simulink model "M10B39_es_V3"  (R2025a)
settings: Solver=ode23tb  StartTime=0.0  StopTime=100  FixedStep=0.001  MaxStep=0.01  RelTol=1e-3  EnableMultiTasking=on
InitFcn:
  | initAll_V3
values from neighbouring files (symbols this model uses):
  acom = 100    [initAll_V1.m]    (also in initAll_V2.m; initAll_V3.m; parameterinit.mat)
  AVm0 = [4.26082678503 4.656135219]    [parameterinit.mat]
  bcom = 50    [initAll_V1.m]    (also in initAll_V2.m; initAll_V3.m; parameterinit.mat)
  commun = 0*commun    [initAll_V1.m]    (also in initAll_V2.m; initAll_V3.m; parameterinit.mat = [0  0  0; 0  0  0; 0  0  0; 0  0  0])
  DataDelay = 0.0*DataDelay    [initAll_V1.m]    (also in initAll_V2.m; initAll_V3.m; parameterinit.mat = [0  0  0; 0  0  0; 0  0  0; 0  0  0])
  ESinit =     [parameterinit.mat]
  fB = 50    [initAll.m]    (also in initAll_V1.m; initAll_V2.m; initAll_V3.m; parameterinit.mat)
  Geninit = Generator_init(opdata,SynMach_in_gidx)    [initAll.m]    (also in initAll_V1.m; initAll_V2.m; initAll_V3.m = Generator_init(opdata_all,SynMach_in_gidx1); parameterinit.mat = )
  lam = 100    [initAll_V1.m]    (also in initAll_V2.m; initAll_V3.m; parameterinit.mat)
  SgridB = 100    [initAll.m]    (also in initAll_V1.m; initAll_V2.m; initAll_V3.m; parameterinit.mat)
  wB = 2*pi*fB    (= 314.159265359)    [initAll.m]    (also in initAll_V1.m; initAll_V2.m; initAll_V3.m; parameterinit.mat)
  Windinit =     [parameterinit.mat]
  YY_load = [3.65450097002 -2.05705688056 0 0 0 0 0 0 0 0 0 0 ... (1521 elements, 39x39)]    [parameterinit.mat]    (also in powerflowcaculate.m = full(YY))
undefined symbols (not defined in the file or in its folder): c1, c2, c3, c4, c5, c6, cp_nom, lambda_nom, P_wind_base, Pelec_base, Pnom
libraries: spsBistableLib x12, simulink_extras x3, slpidlib x2, simulink x1
(part 5 of 7)

== system M10B39_es_V3/Genrators/Wind Generator - DFIG1/Asynchronous Machine Equations  ==
  note: Vsdq
  s / ω_B : Inport
  Vgxy : Inport  Port=2
  Vrxy : Inport  Port=3
  "Trip " : Inport  Port=4
  3th order Transient Equations : Subsystem
  Add : Sum  Inputs=+-
  Constant : Constant  Value=Za
  Constant1 : Constant  Value=0
  Fcn6 : Fcn  Expr=sqrt(u(1)^2+u(2)^2)
  Gain2 : Gain  Gain=NPf
  Interface : Subsystem
  Multiply : Product  Multiplication=Matrix(*)
  Mux2 : Mux  Inputs=2
  Mux4 : Mux  Inputs=2
  Ps_ : Fcn  Expr=u(1)*u(3)+u(2)*u(4)
  Qs_ : Fcn  Expr=u(2)*u(3)-u(1)*u(4)
  Scope : Scope
      settings: ActiveDisplayYMinimum=-0.69793  ActiveDisplayYMaximum=9.95802
  Scope1 : Scope
      settings: ActiveDisplayYMinimum=0.89985  ActiveDisplayYMaximum=1.09985
  Selector : Selector  InputPortWidth=2  IndexOptions=Index vector (dialog)  Indices=[2 1]  OutputSizes=1
  Te_ : Fcn  Expr=u(2)*u(3)+u(1)*u(4)
  Te : Outport
  Ps : Outport  Port=2
  Qs : Outport  Port=3
  Irxy : Outport  Port=4
  Exy : Outport  Port=5
  Isxy1 : Outport  Port=6
  GBxy : Outport  Port=7
  wires:
  "Trip "/1 -> 3th order Transient Equations/4(Trip)
  3th order Transient Equations/1(Irxy) -> Irxy/1
  Qs_/1 -> Qs/1, Scope/1
  Constant1/1 -> Interface/1(delta)
  Gain2/1 -> Te/1
  Vgxy/1 -> Add/1, Fcn6/1, Mux2/1
  Add/1 -> Multiply/2
  Constant/1 -> Multiply/1
  Selector/1 -> Exy/1, Add/2
  Te_/1 -> Gain2/1
  Mux4/1 -> Te_/1
  s / ω_B/1 -> 3th order Transient Equations/3(s / ω_B)
  Ps_/1 -> Ps/1
  Interface/1(Igxy1) -> Isxy1/1
  Interface/2(GBxy) -> GBxy/1
  Mux2/1 -> Qs_/1, Ps_/1
  Vrxy/1 -> 3th order Transient Equations/2(Vrxy)
  Multiply/1 -> 3th order Transient Equations/1(Isxy), Mux4/1, Mux2/2
  Fcn6/1 -> Scope1/1
  3th order Transient Equations/2(Eyx) -> Mux4/2, Selector/1, Interface/2(Eqd)

== system M10B39_es_V3/Genrators/Wind Generator - DFIG1/Converter function ==
  Vsxy : Inport
  Vcxy : Inport  Port=2
  Trip : Inport  Port=3
  Change_choke : Gain  Gain=[1 -1]  SaturateOnIntegerOverflow=on  OutDataTypeStr=Inherit: Same as input  ParamDataTypeStr=Inherit: Same as input
  Constant2 : Constant  Value=0
  GSC_Idq : Integrator  InitialCondition=[Icx0 Icy0]
  L_choke : Gain  Gain=Lg  SaturateOnIntegerOverflow=on  OutDataTypeStr=Inherit: Same as input  ParamDataTypeStr=Inherit: Same as input
  R_choke : Gain  Gain=Rg  SaturateOnIntegerOverflow=on  OutDataTypeStr=Inherit: Same as input  ParamDataTypeStr=Inherit: Same as input
  Selector : Selector  InputPortWidth=2  IndexOptions=Index vector (dialog)  Indices=[2 1]  OutputSizes=1
  Sum : Sum  Inputs=+--+  SaturateOnIntegerOverflow=on
  Switch1 : Switch  Criteria=u2 ~= 0  Threshold=0.5  InputSameDT=off
  Switch4 : Switch  Criteria=u2 ~= 0  Threshold=0.5  InputSameDT=off
  W/L : Gain  Gain=wB / Lg  SaturateOnIntegerOverflow=on  OutDataTypeStr=Inherit: Same as input  ParamDataTypeStr=Inherit: Same as input
  Ixy_gsc : Outport
  wires:
  Switch4/1 -> Ixy_gsc/1, R_choke/1, Selector/1
  GSC_Idq/1 -> Switch4/3
  Switch1/1 -> GSC_Idq/1
  W/L/1 -> Switch1/3
  Constant2/1 -> Switch4/1, Switch1/1
  Trip/1 -> Switch1/2, Switch4/2
  Vcxy/1 -> Sum/2
  Change_choke/1 -> Sum/4
  Sum/1 -> W/L/1
  R_choke/1 -> Sum/3
  Vsxy/1 -> Sum/1
  Selector/1 -> L_choke/1
  L_choke/1 -> Change_choke/1

== system M10B39_es_V3/Genrators/Wind Generator - DFIG1/DC Bus model ==
  note: Pdc = Pr_gsc - Pr_rsc
  Pr_gsc : Inport
  Pr_rsc : Inport  Port=2
  Product2 : Product  Inputs=*/  InputSameDT=on  SaturateOnIntegerOverflow=on  OutDataTypeStr=Inherit: Same as first input
  Sum2 : Sum  Inputs=+-  InputSameDT=on  SaturateOnIntegerOverflow=on  OutDataTypeStr=Inherit: Same as first input
  Udc : Integrator  InitialCondition=Vdc0  LowerSaturationLimit=1e-6  ZeroCross=off
  deg->rad1 : Gain  Gain=1/C_w  SaturateOnIntegerOverflow=on  OutDataTypeStr=Inherit: Same as input  ParamDataTypeStr=Inherit: Same as input
  deg->rad2 : Gain  Gain=wB  SaturateOnIntegerOverflow=on  OutDataTypeStr=Inherit: Same as input  ParamDataTypeStr=Inherit: Same as input
  Vdc : Outport
  wires:
  deg->rad2/1 -> deg->rad1/1
  Sum2/1 -> Product2/1
  deg->rad1/1 -> Udc/1
  Pr_gsc/1 -> Sum2/1
  Product2/1 -> deg->rad2/1  "Idc"
  Udc/1 -> Product2/2, Vdc/1  "Vdc"
  Pr_rsc/1 -> Sum2/2

== system M10B39_es_V3/Genrators/Wind Generator - DFIG1/Grid Side Converter and control ==
  note: K为系数，p/i为系数的名字，DC/Id/Iq为控制的量，g为GSC，w为wind，与直流电网的VSC参数区分开来
  Vdc : Inport
  Vsdq : Inport  Port=2
  Icdq : Inport  Port=3
  Enable : EnablePort
  Add : Sum  Inputs=|+-
  Add{1,3,5,7,11} (5 alike) : Sum
  Add10 : Sum  Commented=on
  Add2 : Sum  Inputs=|+-
  Add4 : Sum  Inputs=|-+
  Add6 : Sum  Inputs=|+-
  Add8 : Sum  Inputs=|-+
  Add9 : Sum  Inputs=-+
  Constant : Constant  Value=Vdc_w
  Constant1 : Constant  Value=Icq_ref
  Constant2 : Constant
  Demux : Demux  Outputs=2
  Demux1 : Demux  Outputs=2
  From12 : From  Commented=on  GotoTag=Icd
  From13 : From  Commented=on  GotoTag=Icq
  From14 : From  Commented=on  GotoTag=Ucd
  From15 : From  Commented=on  GotoTag=Ucq
  Gain : Gain  Gain=KpDC_gw
  Gain1 : Gain  Gain=KiDC_gw
  Gain2 : Gain  Gain=KpId_gw
  Gain3 : Gain  Gain=KiId_gw
  Gain4 : Gain  Gain=Lg
  Gain5 : Gain  Gain=KpIq_gw
  Gain6 : Gain  Gain=KiIq_gw
  Gain7 : Gain  Gain=Lg
  KiDC_gw : Integrator  InitialCondition=Icd_ref
  KiId_gw : Integrator
  KiIq_gw : Integrator
  Multiply{,1,4..5} (4 alike) : Product
  Multiply2 : Product  Commented=on
  Multiply3 : Product  Commented=on
  Mux : Mux  Inputs=2
  Scope1 : Scope
      settings: ActiveDisplayYMinimum=0.114016671  ActiveDisplayYMaximum=0.114016689  DataLoggingVariableName=ScopeData4
  Scope3 : Scope
      settings: ActiveDisplayYMinimum=-1.4E-17  ActiveDisplayYMaximum=9E-18  DataLoggingVariableName=ScopeData11
  Scope4 : Scope
      settings: ActiveDisplayYMinimum=-0.04026  ActiveDisplayYMaximum=0.20394  DataLoggingVariableName=ScopeData12
  Pr_gsc : Outport
  ucdq : Outport  Port=2
  wires:
  Demux1/2 -> [Icq]
  Icdq/1 -> Demux1/1
  Demux1/1 -> [Icd]
  Mux/1 -> ucdq/1
  Add8/1 -> Mux/2
  Add4/1 -> Mux/1
  Add6/1 -> Gain5/1, Gain6/1, Scope3/1
  Add11/1 -> Pr_gsc/1
  Multiply5/1 -> Add11/2
  Multiply4/1 -> Add11/1
  [Vsd] -> Multiply4/1
  [Vsq] -> Multiply5/1
  [Icd] -> Multiply4/2
  [Icq] -> Multiply5/2
  From14/1 -> Multiply2/1
  From12/1 -> Multiply2/2
  Multiply2/1 -> Add10/1
  From15/1 -> Multiply3/1
  From13/1 -> Multiply3/2
  Multiply3/1 -> Add10/2
  Add9/1 -> Add8/2
  Multiply1/1 -> Gain7/1
  [Icd] -> Multiply1/2
  Gain7/1 -> Add9/1
  [Vsq] -> Add9/2
  [We] -> Multiply1/1
  Gain6/1 -> KiIq_gw/1
  Gain5/1 -> Add7/1
  KiIq_gw/1 -> Add7/2
  Add7/1 -> Add8/1  "Vgq'"
  Constant1/1 -> Add6/1
  [Icq] -> Add6/2
  [Vsd] -> Add5/2
  Demux/1 -> [Vsd]
  Demux/2 -> [Vsq]
  Vsdq/1 -> Demux/1, [Vsdq]
  Add5/1 -> Add4/2
  Gain4/1 -> Add5/1
  [Icq] -> Multiply/2
  Multiply/1 -> Gain4/1
  [We] -> Multiply/1
  Add3/1 -> Add4/1  "Vgd'"
  Gain3/1 -> KiId_gw/1
  KiId_gw/1 -> Add3/2
  Add2/1 -> Gain2/1, Gain3/1, Scope4/1
  Gain2/1 -> Add3/1
  [Icd] -> Add2/2, Scope1/1
  Add1/1 -> Add2/1  "Iref_cd*"
  KiDC_gw/1 -> Add1/2
  Gain1/1 -> KiDC_gw/1
  Gain/1 -> Add1/1
  Add/1 -> Gain/1, Gain1/1
  [Vdc] -> Add/2
  Constant/1 -> Add/1
  Constant2/1 -> [We]
  Vdc/1 -> [Vdc]

== system M10B39_es_V3/Genrators/Wind Generator - DFIG1/Mechanical DE ==
  note: 这里是电动机惯例，因此发电的时候力矩应该是负的
  note: $\frac{d\omega_r}{dt}=\frac{1}{H}(T_e-T_m)$
      | 电动机惯例
  Te : Inport
  Tm : Inport  Port=2
  AWr : Integrator  InitialCondition=Wr0
  Add : Sum  Inputs=+-
  Constant2 : Constant
  Gain : Gain  Gain=1/H
  Scope : Scope
      settings: ActiveDisplayYMinimum=0.89006  ActiveDisplayYMaximum=0.98946
  Scope2 : Scope
      settings: ActiveDisplayYMinimum=-0.25  ActiveDisplayYMaximum=2.25  DataLoggingVariableName=ScopeData4
  Sum : Sum  Inputs=|-+
  "s " : Outport
  Wr : Outport  Port=2
  wires:
  Sum/1 -> "s "/1
  Tm/1 -> Scope2/1, Add/2
  Add/1 -> Gain/1
  Constant2/1 -> Sum/2
  Gain/1 -> AWr/1
  Te/1 -> Add/1
  AWr/1 -> Sum/1, Wr/1, Scope/1

== system M10B39_es_V3/Genrators/Wind Generator - DFIG1/NoIdealPLL ==
  note: $-V_{x}*sin(\delta_{pcc})+V_{y}*cos(\delta_{pcc})$
  Vsxy : Inport
  Add : Sum
  Add1 : Sum
  Constant : Constant
  Fcn1 : Fcn  Expr=sqrt(u(1)*u(1)+u(2)*u(2))
  Fcn3 : Fcn  Expr=u(1)*cos(u(3))+u(2)*sin(u(3))
  Fcn4 : Fcn  Expr=-u(1)*sin(u(3))+u(2)*cos(u(3))
  Gain : Gain  Gain=Kppll
  Gain1 : Gain  Gain=Kipll
  Integrator : Integrator
  Mux1 : Mux  Inputs=2
  Mux4 : Mux  Inputs=2
  PLL : Integrator  InitialCondition=Atheta
  Scope{,1..3} (4 alike) : Scope
      Scope settings: ActiveDisplayYMinimum=-0.99937  ActiveDisplayYMaximum=8.99437
      Scope1 settings: ActiveDisplayYMinimum=0.98212  ActiveDisplayYMaximum=1.13956
      Scope2 settings: ActiveDisplayYMinimum=0.98677  ActiveDisplayYMaximum=1.11907  DataLoggingVariableName=ScopeData2
      Scope3 settings: ActiveDisplayYMinimum=0.99657  ActiveDisplayYMaximum=1.01572
  low pass filter : simulink_extras/Additional Linear/Transfer Fcn (with initial outputs)  N=[1]  D="[1e-1  1]"  Y0=1  U0=1
  Vsdq : Outport
  Atheta : Outport  Port=2
  fw : Outport  Port=3
  wires:
  Fcn1/1 -> Scope3/1
  Add1/1 -> PLL/1, Add/1
  Fcn4/1 -> Mux1/2, Gain1/1, Gain/1
  Gain1/1 -> Integrator/1
  Integrator/1 -> Add1/2
  Gain/1 -> Add1/1
  low pass filter/1 -> fw/1, Scope2/1
  Add/1 -> low pass filter/1, Scope1/1
  Constant/1 -> Add/2
  Fcn3/1 -> Mux1/1
  Vsxy/1 -> Mux4/1
  Mux1/1 -> Vsdq/1, Fcn1/1
  Mux4/1 -> Fcn4/1, Fcn3/1
  PLL/1 -> Scope/1, Atheta/1, Mux4/2

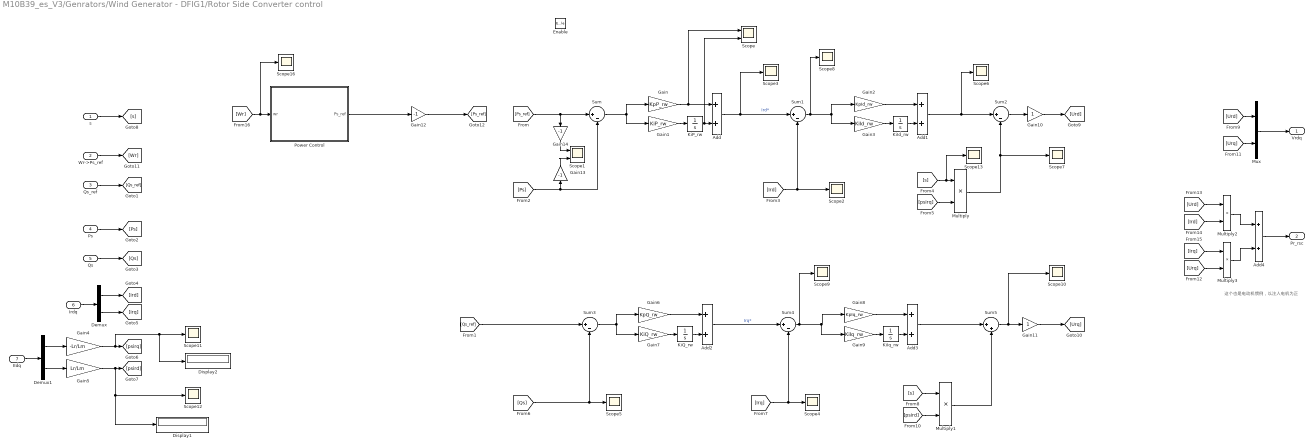
== system M10B39_es_V3/Genrators/Wind Generator - DFIG1/Rotor Side Converter control ==
  note: 这个也是电动机惯例，以注入电机为正
  s : Inport
  Wr->Ps_ref : Inport  Port=2
  Qs_ref : Inport  Port=3
  Ps : Inport  Port=4
  Qs : Inport  Port=5
  Irdq : Inport  Port=6
  Edq : Inport  Port=7
  Enable : EnablePort
  Add{,1..4} (5 alike) : Sum
  Demux : Demux  Outputs=2
  Demux1 : Demux  Outputs=2
  Display1 : Display
  Display2 : Display
  Gain : Gain  Gain=KpP_rw
  Gain1 : Gain  Gain=KiP_rw
  Gain10 : Gain
  Gain11 : Gain
  Gain12 : Gain  Gain=-1
  Gain13 : Gain  Gain=-1
  Gain14 : Gain  Gain=-1
  Gain2 : Gain  Gain=KpId_rw
  Gain3 : Gain  Gain=KiId_rw
  Gain4 : Gain  Gain=-Lr/Lm
  Gain5 : Gain  Gain=Lr/Lm
  Gain6 : Gain  Gain=KpQ_rw
  Gain7 : Gain  Gain=KiQ_rw
  Gain8 : Gain  Gain=KpIq_rw
  Gain9 : Gain  Gain=KiIq_rw
  KiId_rw : Integrator
  KiIq_rw : Integrator
  KiP_rw : Integrator  InitialCondition=Ird_ref
  KiQ_rw : Integrator  InitialCondition=Irq_ref
  Multiply{,1..3} (4 alike) : Product
  Mux : Mux  Inputs=2
  Power Control : Subsystem
  Scope : Scope  NumInputPorts=2
      settings: ActiveDisplayYMinimum=-0.15787  ActiveDisplayYMaximum=1.4048
  Scope1 : Scope  NumInputPorts=2
      settings: ActiveDisplayYMinimum=0.941157  ActiveDisplayYMaximum=0.94124  DataLoggingVariableName=ScopeData2
  Scope{2..13,16} (13 alike) : Scope
      Scope10 settings: ActiveDisplayYMinimum=-0.02713  ActiveDisplayYMaximum=0.00724  DataLoggingVariableName=ScopeData10
      Scope11 settings: DataLoggingVariableName=ScopeData13
      Scope12 settings: DataLoggingVariableName=ScopeData14
      Scope13 settings: ActiveDisplayYMinimum=-0.23407  ActiveDisplayYMaximum=0.19201  DataLoggingVariableName=ScopeData15
      Scope16 settings: ActiveDisplayYMinimum=-1.125  ActiveDisplayYMaximum=0.125  DataLoggingVariableName=ScopeData2
      Scope2 settings: ActiveDisplayYMinimum=0.9164  ActiveDisplayYMaximum=0.98721  DataLoggingVariableName=ScopeData4
      Scope3 settings: ActiveDisplayYMinimum=1.1610912356  ActiveDisplayYMaximum=1.1610912369  DataLoggingVariableName=ScopeData5
      Scope4 settings: ActiveDisplayYMinimum=-0.86275  ActiveDisplayYMaximum=6.60838  DataLoggingVariableName=ScopeData2
      Scope5 settings: ActiveDisplayYMinimum=-8E-13  ActiveDisplayYMaximum=6E-13  DataLoggingVariableName=ScopeData3
      Scope6 settings: ActiveDisplayYMinimum=0.00428  ActiveDisplayYMaximum=0.05974  DataLoggingVariableName=ScopeData2
      Scope7 settings: ActiveDisplayYMinimum=-0.10258  ActiveDisplayYMaximum=-0.10236  DataLoggingVariableName=ScopeData3
      Scope8 settings: ActiveDisplayYMinimum=-0.15319  ActiveDisplayYMaximum=1.32201  DataLoggingVariableName=ScopeData4
      Scope9 settings: ActiveDisplayYMinimum=-0.42548  ActiveDisplayYMaximum=0.04779  DataLoggingVariableName=ScopeData9
  Sum{,1..4} (5 alike) : Sum  Inputs=|+-
  Sum5 : Sum  Inputs=|++
  Vrdq : Outport
  Pr_rsc : Outport  Port=2
  wires:
  Gain12/1 -> [Ps_ref]
  Gain13/1 -> Scope1/2
  Gain14/1 -> Scope1/1
  [Qs_ref] -> Sum3/1
  Power Control/1(Ps_ref) -> Gain12/1
  [Wr] -> Power Control/1(wr), Scope16/1
  [Ird] -> Sum1/2, Scope2/1
  Add4/1 -> Pr_rsc/1
  Multiply3/1 -> Add4/2
  Multiply2/1 -> Add4/1
  [Urq] -> Multiply3/2
  [Irq] -> Multiply3/1
  [Ird] -> Multiply2/2
  [Urd] -> Multiply2/1
  KiP_rw/1 -> Add/2, Scope/2
  Gain/1 -> Add/1, Scope/1
  Gain11/1 -> [Urq]
  Gain10/1 -> [Urd]
  Mux/1 -> Vrdq/1
  [Urq] -> Mux/2
  [Urd] -> Mux/1
  Sum5/1 -> Gain11/1, Scope10/1
  Multiply1/1 -> Sum5/2
  [psird] -> Multiply1/2
  [s] -> Multiply1/1
  Add3/1 -> Sum5/1
  Gain9/1 -> KiIq_rw/1
  Sum4/1 -> Gain8/1, Gain9/1, Scope9/1
  Gain8/1 -> Add3/1
  KiIq_rw/1 -> Add3/2
  [Irq] -> Sum4/2, Scope4/1
  Gain7/1 -> KiQ_rw/1
  KiQ_rw/1 -> Add2/2
  Gain6/1 -> Add2/1
  Sum3/1 -> Gain6/1, Gain7/1
  Add2/1 -> Sum4/1  "Irq*"
  [Qs] -> Sum3/2, Scope5/1
  Sum2/1 -> Gain10/1
  Multiply/1 -> Sum2/2, Scope7/1
  [psirq] -> Multiply/2
  [s] -> Multiply/1, Scope13/1
  Gain5/1 -> [psird], Display1/1, Scope12/1
  Gain4/1 -> [psirq], Scope11/1, Display2/1
  Demux1/1 -> Gain4/1
  s/1 -> [s]
  Edq/1 -> Demux1/1
  Demux1/2 -> Gain5/1
  Gain3/1 -> KiId_rw/1
  KiId_rw/1 -> Add1/2
  Gain2/1 -> Add1/1
  Sum1/1 -> Gain2/1, Gain3/1, Scope8/1
  Add1/1 -> Sum2/1, Scope6/1
  Add/1 -> Scope3/1, Sum1/1  "Ird*"
  Sum/1 -> Gain/1, Gain1/1
  Gain1/1 -> KiP_rw/1
  [Ps] -> Gain13/1, Sum/2
  [Ps_ref] -> Sum/1, Gain14/1
  Demux/2 -> [Irq]
  Demux/1 -> [Ird]
  Irdq/1 -> Demux/1
  Qs/1 -> [Qs]
  Ps/1 -> [Ps]
  Qs_ref/1 -> [Qs_ref]
  Wr->Ps_ref/1 -> [Wr]

== system M10B39_es_V3/Genrators/Wind Generator - DFIG1/Wind Turbine ==
  note: $C_p=0.22* \lbrack 116*(\frac{1}{\lambda+0.008\beta}-\frac{0.0035}{\beta^3+1})-0.48\beta-5 \rbrack * e^{-12.5*(\frac{1}{\lambda+0.08\beta}-\frac{0.035}{\beta^3+1}) }$
  note: $P_m=0.95*\frac{1.2}{(12^3*0.5)}*\lbrack 43.268*(\frac{v_w}{99.4945*\omega_r}-0.035)-1.865 \rbrack * e^{-12.5*(\frac{v_w}{99.4945*\omega_r}-0.035) }*v_w^3$
  note: $C_p= \lbrack 43.268*(\frac{v_w}{99.4945*\omega_r}-0.035)-1.865 \rbrack * e^{-12.5*(\frac{v_w}{99.4945*\omega_r}-0.035) }$
  note: $P_m=0.95*\frac{1.2}{(12^3*0.5)}*\lbrack 43.268*(\frac{1}{99.4945*\frac{\omega_r}{v_w}}-0.035)-1.865 \rbrack * e^{-12.5*(\frac{1}{99.4945*\frac{\omega_r}{v_w}}-0.035) }*v_w^3$
  note: $C_p= \lbrack 43.268*(\frac{1}{99.4945*\frac{\omega_r}{v_w}}-0.035)-1.865 \rbrack * e^{-12.5*(\frac{1}{99.4945*\frac{\omega_r}{v_w}}-0.035) }$
  note: $P_m=0.95*\frac{1.2}{(12^3*0.5)}*C_p*v_w^3$
  note: $C_p= \lbrack 43.268*(\frac{1}{\lambda}-0.035)-1.865 \rbrack * e^{-12.5*(\frac{1}{\lambda}-0.035) }$
  note: $C_p=0.373* \lbrack 116*(\frac{1}{\lambda}-0.035)-5 \rbrack * e^{-12.5*(\frac{1}{\lambda}-0.035) }$
  note: 叶片旋转角速度
  note: 风力机输出
      | 的机械功率
  note: 叶尖速比
  note: 风能利用系数与桨矩角
      | 和叶尖速比之间的关系
  note: 风能利用
      | 系数
  note: 风力机输出
      | 的机械功率
  note: 风速
  note: 叶片旋转速度
  note: 考虑了机械损耗
  note: $\lambda=99.4945*\frac{\omega_r}{v_w}$
  note: $C_p=0.373* \lbrack 116*(\frac{1}{\lambda+0.08\beta}-\frac{0.035}{\beta^3+1})-0.4\beta-5 \rbrack * e^{-12.5*(\frac{1}{\lambda+0.08\beta}-\frac{0.035}{\beta^3+1}) }$
  note: $P_m=\frac{1.2}{(12^3*0.5)}*C_p*v_w^3$
  note: J. Chen and D. Jiang, "Study on modeling and simulation of non-grid-connected wind turbine," 2009 World Non-Grid-Connected Wind Power and Energy Conference , Nanjing, 2009, pp. 1-5. doi: 10.1109/WNWEC.2009.5335791
  W_wt (pu) : Inport
  Pitch angle (deg) : Inport  Port=2
  Wind speed (m/s) : Inport  Port=3
  ->pu1 : Gain  Gain=0.95
  ->pu2 : Gain  Gain=0.95
  Avoid div. by zero : Saturate  UpperLimit=inf  LowerLimit=eps
  "Avoid div. by zero " : Saturate  UpperLimit=inf  LowerLimit=eps
  Display2 : Display
  Fcn2 : Fcn  Expr=99.4945*u[2]/u[1]
  Fcn4 : Fcn  Expr=0.22*(116*(1/(u(1)+0.008*u(2))-0.0035/((u(2)^3)+1))-0.48*u(2)-5)*exp(-12.5*(1/(u(1)+0.008*u(2))-0.0035/((u(2)^3)+1)))
  "K2*Cp*wind^3 " : Fcn  Expr=1.2/(12^3*0.5)*u[1]^3*u[2]
  Mux : Mux  Inputs=2
  Mux1 : Mux  Inputs=2
  Mux2 : Mux  Inputs=2
  Product2 : Product  Inputs=*/  InputSameDT=on  SaturateOnIntegerOverflow=on  OutDataTypeStr=Inherit: Same as first input
  Scope{1..3,5} (4 alike) : Scope
      Scope1 settings: ActiveDisplayYMinimum=6.3327  ActiveDisplayYMaximum=6.33385  DataLoggingSaveFormat=Array
      Scope2 settings: ActiveDisplayYMinimum=0.10425  ActiveDisplayYMaximum=1.46932  DataLoggingVariableName=ScopeData25
      Scope3 settings: ActiveDisplayYMinimum=0.5999  ActiveDisplayYMaximum=0.6001  DataLoggingVariableName=Pw  DataLoggingSaveFormat=Array
      Scope5 settings: ActiveDisplayYMinimum=0.64296  ActiveDisplayYMaximum=0.84296  DataLoggingVariableName=Pw2  DataLoggingSaveFormat=Array
  Subsystem : Subsystem  Commented=on
  Tm : Outport
  Pm : Outport  Port=2
  wires:
  ->pu2/1 -> Pm/1
  Fcn4/1 -> Scope5/1, Mux2/2
  "K2*Cp*wind^3 "/1 -> Scope3/1, Display2/1, Product2/1, ->pu2/1
  Wind speed (m/s)/1 -> Avoid div. by zero/1
  Product2/1 -> ->pu1/1
  ->pu1/1 -> Scope2/1, Tm/1
  W_wt (pu)/1 -> "Avoid div. by zero "/1
  "Avoid div. by zero "/1 -> Product2/2, Mux/2
  Avoid div. by zero/1 -> Mux2/1, Mux/1
  Pitch angle (deg)/1 -> Mux1/2
  Mux2/1 -> "K2*Cp*wind^3 "/1
  Mux/1 -> Fcn2/1
  Mux1/1 -> Fcn4/1
  Fcn2/1 -> Mux1/1, Scope1/1  "lambda"

== system M10B39_es_V3/Genrators/Wind Generator - DFIG1/dq-xy ==
  dq : Inport
  delta_xy : Inport  Port=2
  Complex to Magnitude-Angle : ComplexToMagnitudeAngle
  Demux : Demux  Outputs=2
  Fcn3 : Fcn  Expr=u(1)*cos(u(2))
  Fcn4 : Fcn  Expr=u(1)*sin(u(2))
  Mux1 : Mux  Inputs=2
  Mux2 : Mux  Inputs=2
  Real-Imag to Complex : RealImagToComplex
  Scope : Scope
      settings: ActiveDisplayYMinimum=0.298155365983  ActiveDisplayYMaximum=0.298155366015  DataLoggingVariableName=ScopeData2
  Scope1 : Scope  NumInputPorts=2
      settings: ActiveDisplayYMinimum=1.04058  ActiveDisplayYMaximum=1.12593  DataLoggingVariableName=ScopeData51  DataLoggingSaveFormat=Array
  Scope2 : Scope  NumInputPorts=2
      settings: ActiveDisplayYMinimum=1.01502  ActiveDisplayYMaximum=1.10979  DataLoggingVariableName=ScopeData56  DataLoggingSaveFormat=Array
  Sum14 : Sum  Inputs=|++
  xy : Outport
  wires:
  Mux2/1 -> xy/1
  dq/1 -> Demux/1
  Demux/2 -> Real-Imag to Complex/2
  Demux/1 -> Real-Imag to Complex/1
  Real-Imag to Complex/1 -> Complex to Magnitude-Angle/1
  delta_xy/1 -> Sum14/2
  Fcn3/1 -> Mux2/1, Scope2/1
  Fcn4/1 -> Scope2/2, Mux2/2
  Mux1/1 -> Fcn3/1, Fcn4/1
  Complex to Magnitude-Angle/2 -> Sum14/1, Scope/1
  Complex to Magnitude-Angle/1 -> Mux1/1, Scope1/1
  Sum14/1 -> Mux1/2, Scope1/2

== system M10B39_es_V3/Genrators/Wind Generator - DFIG1/dq-xy1 ==
  dq : Inport
  delta_xy : Inport  Port=2
  Complex to Magnitude-Angle : ComplexToMagnitudeAngle
  Demux : Demux  Outputs=2
  Fcn3 : Fcn  Expr=u(1)*cos(u(2))
  Fcn4 : Fcn  Expr=u(1)*sin(u(2))
  Mux1 : Mux  Inputs=2
  Mux2 : Mux  Inputs=2
  Real-Imag to Complex : RealImagToComplex
  Scope : Scope
      settings: ActiveDisplayYMinimum=0.298155365983  ActiveDisplayYMaximum=0.298155366015  DataLoggingVariableName=ScopeData2
  Scope1 : Scope  NumInputPorts=2
      settings: ActiveDisplayYMinimum=1.04058  ActiveDisplayYMaximum=1.12593  DataLoggingVariableName=ScopeData51  DataLoggingSaveFormat=Array
  Scope2 : Scope  NumInputPorts=2
      settings: ActiveDisplayYMinimum=1.01502  ActiveDisplayYMaximum=1.10979  DataLoggingVariableName=ScopeData56  DataLoggingSaveFormat=Array
  Sum14 : Sum  Inputs=|++
  xy : Outport
  wires:
  Mux2/1 -> xy/1
  dq/1 -> Demux/1
  Demux/2 -> Real-Imag to Complex/2
  Demux/1 -> Real-Imag to Complex/1
  Real-Imag to Complex/1 -> Complex to Magnitude-Angle/1
  delta_xy/1 -> Sum14/2
  Fcn3/1 -> Mux2/1, Scope2/1
  Fcn4/1 -> Scope2/2, Mux2/2
  Mux1/1 -> Fcn3/1, Fcn4/1
  Complex to Magnitude-Angle/2 -> Sum14/1, Scope/1
  Complex to Magnitude-Angle/1 -> Mux1/1, Scope1/1
  Sum14/1 -> Mux1/2, Scope1/2

== system M10B39_es_V3/Genrators/Wind Generator - DFIG1/help ==
  note: $P_m=0.95*\frac{1.2}{(12^3*0.5)}*\lbrack 43.268*(\frac{v_w}{99.4945*\omega_r}-0.035)-1.865 \rbrack * e^{-12.5*(\frac{v_w}{99.4945*\omega_r}-0.035) }*v_w^3$
  note: $P_w=P_m=(1-s)*P_s=\omega_r*2*(0.5*\omega_r^2+0.05*\omega_r+0.12)$
  note: $P_s^{ref}=2*(0.5000*\omega_r^2+0.0500*\omega_r+0.1200)$
  note: 从诺顿支路的角度考虑，VSC可以等效成纯的电流源，与等效成诺顿支路的异步电机的虚拟电流应该是可以直接相加
      | 现在关键问题是，异步电机的虚拟电流已经转换成了xy坐标系下的量。
      | 我下面要证明
      | 异步电机实际电流Igxy+VSC实际电流Icxy= [（异步电机实际电流Igdq+VSC实际电流Icdq）-->xy]
  note: $I_{gxy}+I_{cxy}\\ =[-I_{gxy}^{\prime}+(ZP)^{-1}PV_{gxy}]+I_{cxy}$
  note: $-I_{sdq}=I_{sdq}^{\prime}-Z^{-1}V_{sdq}\\ 其中I_{sdq}^{\prime}=Z^{-1}E_{dq}$
  note: 可以看到完全一致，在模型中可以先变Icdq为Icxy，再与虚拟电流xy相加
  note: $I_{gxy}+I_{cxy}\\ =[-I_{gxy}^{\prime}+(ZP)^{-1}PV_{gxy}]+I_{cxy}$
  note: $PV_{sxy}=E_{dq}+ZPI_{sxy}$
  note: $\pmatrix{A_d \cr A_q}=\pmatrix{cos\theta & sin\theta \cr -sin\theta & cos\theta}\pmatrix{A_x \cr A_y}\\ P=\pmatrix{cos\theta & sin\theta \cr -sin\theta & cos\theta}$
  note: $(ZP)^{-1}PV_{sxy}=(ZP)^{-1}E_{dq}+I_{sxy}$
  note: $-I_{sxy}=(ZP)^{-1}E_{dq}-(ZP)^{-1}PV_{sxy}$
  note: $A_{dq}=PA_{xy}\\ A_{xy}=P^{-1}A_{dq}$
  note: $-I_{sxy}=I_{sxy}^{\prime}-(ZP)^{-1}PV_{sxy}\\ 其中I_{sxy}^{\prime}=(ZP)^{-1}E_{dq}$
  note: $V_{sdq}=E_{dq}+ZI_{sdq}$
  note: $-I_{sdq}=Z^{-1}E_{dq}-Z^{-1}V_{sdq}$
  note: $V_{sdq}=E_{dq}+ZI_{sdq}$
  note: $PI_{gxy}+PI_{cxy}\\ =[-PI_{gxy}^{\prime}+Z^{-1}PV_{gxy}]+PI_{cxy}$
  note: $I_{gxy}+I_{cxy}\\ =[-I_{gxy}^{\prime}+P^{-1}Z^{-1}PV_{gxy}]+I_{cxy}$
  note: $I_{gdq}+I_{cdq}\\ =[-I_{gdq}^{\prime}+Z^{-1}V_{gdq}]+I_{cdq}$
  note: $Z^{-1}V_{sdq}=Z^{-1}E_{dq}+I_{sdq}$
  note: $\omega_{r}=(1-s)*\omega_1$

== system M10B39_es_V3/Genrators/Wind Generator - DFIG1/output ==
  Isxy1 : Inport
  Ixy_gsc : Inport  Port=2
  GB : Inport  Port=3
  Ps : Inport  Port=4
  Prgsc : Inport  Port=5
  fw : Inport  Port=6
  Wr : Inport  Port=7
  Add : Sum
  Add1 : Sum
  Bus Creator : BusCreator  Inputs=3
  Demux : Demux
  Gain2 : Gain  Gain=SwgeqB./SgridB
  Gain3 : Gain
  Gain4 : Gain
  Gain5 : Gain  Gain=-1
  Gain6 : Gain  Gain=SwgeqB./SgridB
  Gain7 : Gain  Gain=-1
  Gain8 : Gain  Gain=SwgeqB./SgridB
  Scope : Scope  NumInputPorts=4
      settings: ActiveDisplayYMinimum=-54.46215  ActiveDisplayYMaximum=-34.46215  DataLoggingVariableName=ScopeData5
  Scope{4..5,7..8} (4 alike) : Scope
      Scope4 settings: ActiveDisplayYMinimum=-50.97357  ActiveDisplayYMaximum=11.3279  DataLoggingVariableName=ScopeData4
      Scope5 settings: TimeSpan=200  ActiveDisplayYMinimum=0.47861  ActiveDisplayYMaximum=6.19543  DataLoggingVariableName=ScopeData6
      Scope7 settings: ActiveDisplayYMinimum=-2.00383  ActiveDisplayYMaximum=-0.83205  DataLoggingVariableName=ScopeData7
      Scope8 settings: ActiveDisplayYMinimum=-0.15764  ActiveDisplayYMaximum=0.7029  DataLoggingVariableName=ScopeData8
  m : Outport
  Igxy : Outport  Port=2
  GBxy : Outport  Port=3
  wires:
  Wr/1 -> Bus Creator/3  "Wr"
  fw/1 -> Bus Creator/2  "fw"
  Bus Creator/1 -> m/1
  Ps/1 -> Add1/1, Scope7/1
  Add1/1 -> Gain7/1
  Gain7/1 -> Gain8/1
  Gain8/1 -> Bus Creator/1, Scope5/1  "Pwind"
  Prgsc/1 -> Add1/2, Scope8/1
  GB/1 -> Gain3/1
  Gain3/1 -> Gain6/1
  Gain6/1 -> GBxy/1, Demux/1
  Demux/3 -> Scope/3
  Demux/4 -> Scope/4
  Demux/1 -> Scope/1
  Demux/2 -> Scope/2
  Gain5/1 -> Add/2
  Gain4/1 -> Add/1
  Ixy_gsc/1 -> Gain5/1
  Add/1 -> Gain2/1
  Gain2/1 -> Scope4/1, Igxy/1
  Isxy1/1 -> Gain4/1

== system M10B39_es_V3/Genrators/Wind Generator - DFIG1/xy->dq1 ==
  Ixy : Inport
  Theta : Inport  Port=2
  Complex to Magnitude-Angle : ComplexToMagnitudeAngle
  Complex to Real-Imag : ComplexToRealImag
  Demux1 : Demux  Outputs=2
      settings: DisplayOption=none
  Magnitude-Angle to Complex : MagnitudeAngleToComplex
  Mux : Mux  Inputs=2
  Real-Imag to Complex : RealImagToComplex
  Scope : Scope
      settings: ActiveDisplayYMinimum=3.11918  ActiveDisplayYMaximum=3.16079
  Scope1 : Scope
      settings: ActiveDisplayYMinimum=2.59405  ActiveDisplayYMaximum=3.13201  DataLoggingVariableName=ScopeData3
  Sum1 : Sum  Inputs=|+-  SaturateOnIntegerOverflow=on
  Idq : Outport
  wires:
  Complex to Magnitude-Angle/1 -> Magnitude-Angle to Complex/1
  Theta/1 -> Sum1/2
  Complex to Magnitude-Angle/2 -> Sum1/1, Scope1/1
  Demux1/1 -> Real-Imag to Complex/1
  Complex to Real-Imag/2 -> Mux/2  "Iq"
  Mux/1 -> Idq/1
  Complex to Real-Imag/1 -> Mux/1  "Id"
  Magnitude-Angle to Complex/1 -> Complex to Real-Imag/1
  Sum1/1 -> Magnitude-Angle to Complex/2, Scope/1
  Demux1/2 -> Real-Imag to Complex/2
  Real-Imag to Complex/1 -> Complex to Magnitude-Angle/1
  Ixy/1 -> Demux1/1

== system M10B39_es_V3/Genrators/Wind Generator - DFIG1/xy->dq2 ==
  Ixy : Inport
  Theta : Inport  Port=2
  Complex to Magnitude-Angle : ComplexToMagnitudeAngle
  Complex to Real-Imag : ComplexToRealImag
  Demux1 : Demux  Outputs=2
      settings: DisplayOption=none
  Magnitude-Angle to Complex : MagnitudeAngleToComplex
  Mux : Mux  Inputs=2
  Real-Imag to Complex : RealImagToComplex
  Scope : Scope
      settings: ActiveDisplayYMinimum=3.11918  ActiveDisplayYMaximum=3.16079
  Scope1 : Scope
      settings: ActiveDisplayYMinimum=2.59405  ActiveDisplayYMaximum=3.13201  DataLoggingVariableName=ScopeData3
  Sum1 : Sum  Inputs=|+-  SaturateOnIntegerOverflow=on
  Idq : Outport
  wires:
  Complex to Magnitude-Angle/1 -> Magnitude-Angle to Complex/1
  Theta/1 -> Sum1/2
  Complex to Magnitude-Angle/2 -> Sum1/1, Scope1/1
  Demux1/1 -> Real-Imag to Complex/1
  Complex to Real-Imag/2 -> Mux/2  "Iq"
  Mux/1 -> Idq/1
  Complex to Real-Imag/1 -> Mux/1  "Id"
  Magnitude-Angle to Complex/1 -> Complex to Real-Imag/1
  Sum1/1 -> Magnitude-Angle to Complex/2, Scope/1
  Demux1/2 -> Real-Imag to Complex/2
  Real-Imag to Complex/1 -> Complex to Magnitude-Angle/1
  Ixy/1 -> Demux1/1

== system M10B39_es_V3/Genrators/Wind Generator - DFIG1/xy->dq3 ==
  Ixy : Inport
  Theta : Inport  Port=2
  Complex to Magnitude-Angle : ComplexToMagnitudeAngle
  Complex to Real-Imag : ComplexToRealImag
  Demux1 : Demux  Outputs=2
      settings: DisplayOption=none
  Magnitude-Angle to Complex : MagnitudeAngleToComplex
  Mux : Mux  Inputs=2
  Real-Imag to Complex : RealImagToComplex
  Scope : Scope
      settings: ActiveDisplayYMinimum=3.11918  ActiveDisplayYMaximum=3.16079
  Scope1 : Scope
      settings: ActiveDisplayYMinimum=2.59405  ActiveDisplayYMaximum=3.13201  DataLoggingVariableName=ScopeData3
  Sum1 : Sum  Inputs=|+-  SaturateOnIntegerOverflow=on
  Idq : Outport
  wires:
  Complex to Magnitude-Angle/1 -> Magnitude-Angle to Complex/1
  Theta/1 -> Sum1/2
  Complex to Magnitude-Angle/2 -> Sum1/1, Scope1/1
  Demux1/1 -> Real-Imag to Complex/1
  Complex to Real-Imag/2 -> Mux/2  "Iq"
  Mux/1 -> Idq/1
  Complex to Real-Imag/1 -> Mux/1  "Id"
  Magnitude-Angle to Complex/1 -> Complex to Real-Imag/1
  Sum1/1 -> Magnitude-Angle to Complex/2, Scope/1
  Demux1/2 -> Real-Imag to Complex/2
  Real-Imag to Complex/1 -> Complex to Magnitude-Angle/1
  Ixy/1 -> Demux1/1

== system M10B39_es_V3/Genrators/Wind Generator - DFIG2/Asynchronous Machine Equations  ==
  note: Vsdq
  s / ω_B : Inport
  Vgxy : Inport  Port=2
  Vrxy : Inport  Port=3
  "Trip " : Inport  Port=4
  3th order Transient Equations : Subsystem
  Add : Sum  Inputs=+-
  Constant : Constant  Value=Za
  Constant1 : Constant  Value=0
  Fcn6 : Fcn  Expr=sqrt(u(1)^2+u(2)^2)
  Gain2 : Gain  Gain=NPf
  Interface : Subsystem
  Multiply : Product  Multiplication=Matrix(*)
  Mux2 : Mux  Inputs=2
  Mux4 : Mux  Inputs=2
  Ps_ : Fcn  Expr=u(1)*u(3)+u(2)*u(4)
  Qs_ : Fcn  Expr=u(2)*u(3)-u(1)*u(4)
  Scope : Scope
      settings: ActiveDisplayYMinimum=-0.69793  ActiveDisplayYMaximum=9.95802
  Scope1 : Scope
      settings: ActiveDisplayYMinimum=0.89985  ActiveDisplayYMaximum=1.09985
  Selector : Selector  InputPortWidth=2  IndexOptions=Index vector (dialog)  Indices=[2 1]  OutputSizes=1
  Te_ : Fcn  Expr=u(2)*u(3)+u(1)*u(4)
  Te : Outport
  Ps : Outport  Port=2
  Qs : Outport  Port=3
  Irxy : Outport  Port=4
  Exy : Outport  Port=5
  Isxy1 : Outport  Port=6
  GBxy : Outport  Port=7
  wires:
  "Trip "/1 -> 3th order Transient Equations/4(Trip)
  3th order Transient Equations/1(Irxy) -> Irxy/1
  Qs_/1 -> Qs/1, Scope/1
  Constant1/1 -> Interface/1(delta)
  Gain2/1 -> Te/1
  Vgxy/1 -> Add/1, Fcn6/1, Mux2/1
  Add/1 -> Multiply/2
  Constant/1 -> Multiply/1
  Selector/1 -> Exy/1, Add/2
  Te_/1 -> Gain2/1
  Mux4/1 -> Te_/1
  s / ω_B/1 -> 3th order Transient Equations/3(s / ω_B)
  Ps_/1 -> Ps/1
  Interface/1(Igxy1) -> Isxy1/1
  Interface/2(GBxy) -> GBxy/1
  Mux2/1 -> Qs_/1, Ps_/1
  Vrxy/1 -> 3th order Transient Equations/2(Vrxy)
  Multiply/1 -> 3th order Transient Equations/1(Isxy), Mux4/1, Mux2/2
  Fcn6/1 -> Scope1/1
  3th order Transient Equations/2(Eyx) -> Mux4/2, Selector/1, Interface/2(Eqd)

== system M10B39_es_V3/Genrators/Wind Generator - DFIG2/Converter function ==
  Vsxy : Inport
  Vcxy : Inport  Port=2
  Trip : Inport  Port=3
  Change_choke : Gain  Gain=[1 -1]  SaturateOnIntegerOverflow=on  OutDataTypeStr=Inherit: Same as input  ParamDataTypeStr=Inherit: Same as input
  Constant2 : Constant  Value=0
  GSC_Idq : Integrator  InitialCondition=[Icx0 Icy0]
  L_choke : Gain  Gain=Lg  SaturateOnIntegerOverflow=on  OutDataTypeStr=Inherit: Same as input  ParamDataTypeStr=Inherit: Same as input
  R_choke : Gain  Gain=Rg  SaturateOnIntegerOverflow=on  OutDataTypeStr=Inherit: Same as input  ParamDataTypeStr=Inherit: Same as input
  Selector : Selector  InputPortWidth=2  IndexOptions=Index vector (dialog)  Indices=[2 1]  OutputSizes=1
  Sum : Sum  Inputs=+--+  SaturateOnIntegerOverflow=on
  Switch1 : Switch  Criteria=u2 ~= 0  Threshold=0.5  InputSameDT=off
  Switch4 : Switch  Criteria=u2 ~= 0  Threshold=0.5  InputSameDT=off
  W/L : Gain  Gain=wB / Lg  SaturateOnIntegerOverflow=on  OutDataTypeStr=Inherit: Same as input  ParamDataTypeStr=Inherit: Same as input
  Ixy_gsc : Outport
  wires:
  Switch4/1 -> Ixy_gsc/1, R_choke/1, Selector/1
  GSC_Idq/1 -> Switch4/3
  Switch1/1 -> GSC_Idq/1
  W/L/1 -> Switch1/3
  Constant2/1 -> Switch4/1, Switch1/1
  Trip/1 -> Switch1/2, Switch4/2
  Vcxy/1 -> Sum/2
  Change_choke/1 -> Sum/4
  Sum/1 -> W/L/1
  R_choke/1 -> Sum/3
  Vsxy/1 -> Sum/1
  Selector/1 -> L_choke/1
  L_choke/1 -> Change_choke/1

== system M10B39_es_V3/Genrators/Wind Generator - DFIG2/DC Bus model ==
  note: Pdc = Pr_gsc - Pr_rsc
  Pr_gsc : Inport
  Pr_rsc : Inport  Port=2
  Product2 : Product  Inputs=*/  InputSameDT=on  SaturateOnIntegerOverflow=on  OutDataTypeStr=Inherit: Same as first input
  Sum2 : Sum  Inputs=+-  InputSameDT=on  SaturateOnIntegerOverflow=on  OutDataTypeStr=Inherit: Same as first input
  Udc : Integrator  InitialCondition=Vdc0  LowerSaturationLimit=1e-6  ZeroCross=off
  deg->rad1 : Gain  Gain=1/C_w  SaturateOnIntegerOverflow=on  OutDataTypeStr=Inherit: Same as input  ParamDataTypeStr=Inherit: Same as input
  deg->rad2 : Gain  Gain=wB  SaturateOnIntegerOverflow=on  OutDataTypeStr=Inherit: Same as input  ParamDataTypeStr=Inherit: Same as input
  Vdc : Outport
  wires:
  deg->rad2/1 -> deg->rad1/1
  Sum2/1 -> Product2/1
  deg->rad1/1 -> Udc/1
  Pr_gsc/1 -> Sum2/1
  Product2/1 -> deg->rad2/1  "Idc"
  Udc/1 -> Product2/2, Vdc/1  "Vdc"
  Pr_rsc/1 -> Sum2/2

== system M10B39_es_V3/Genrators/Wind Generator - DFIG2/Grid Side Converter and control ==
  note: K为系数，p/i为系数的名字，DC/Id/Iq为控制的量，g为GSC，w为wind，与直流电网的VSC参数区分开来
  Vdc : Inport
  Vsdq : Inport  Port=2
  Icdq : Inport  Port=3
  Enable : EnablePort
  Add : Sum  Inputs=|+-
  Add{1,3,5,7,11} (5 alike) : Sum
  Add10 : Sum  Commented=on
  Add2 : Sum  Inputs=|+-
  Add4 : Sum  Inputs=|-+
  Add6 : Sum  Inputs=|+-
  Add8 : Sum  Inputs=|-+
  Add9 : Sum  Inputs=-+
  Constant : Constant  Value=Vdc_w
  Constant1 : Constant  Value=Icq_ref
  Constant2 : Constant
  Demux : Demux  Outputs=2
  Demux1 : Demux  Outputs=2
  From12 : From  Commented=on  GotoTag=Icd
  From13 : From  Commented=on  GotoTag=Icq
  From14 : From  Commented=on  GotoTag=Ucd
  From15 : From  Commented=on  GotoTag=Ucq
  Gain : Gain  Gain=KpDC_gw
  Gain1 : Gain  Gain=KiDC_gw
  Gain2 : Gain  Gain=KpId_gw
  Gain3 : Gain  Gain=KiId_gw
  Gain4 : Gain  Gain=Lg
  Gain5 : Gain  Gain=KpIq_gw
  Gain6 : Gain  Gain=KiIq_gw
  Gain7 : Gain  Gain=Lg
  KiDC_gw : Integrator  InitialCondition=Icd_ref
  KiId_gw : Integrator
  KiIq_gw : Integrator
  Multiply{,1,4..5} (4 alike) : Product
  Multiply2 : Product  Commented=on
  Multiply3 : Product  Commented=on
  Mux : Mux  Inputs=2
  Scope1 : Scope
      settings: ActiveDisplayYMinimum=0.114016671  ActiveDisplayYMaximum=0.114016689  DataLoggingVariableName=ScopeData4
  Scope3 : Scope
      settings: ActiveDisplayYMinimum=-1.4E-17  ActiveDisplayYMaximum=9E-18  DataLoggingVariableName=ScopeData11
  Scope4 : Scope
      settings: ActiveDisplayYMinimum=-0.04026  ActiveDisplayYMaximum=0.20394  DataLoggingVariableName=ScopeData12
  Pr_gsc : Outport
  ucdq : Outport  Port=2
  wires:
  Demux1/2 -> [Icq]
  Icdq/1 -> Demux1/1
  Demux1/1 -> [Icd]
  Mux/1 -> ucdq/1
  Add8/1 -> Mux/2
  Add4/1 -> Mux/1
  Add6/1 -> Gain5/1, Gain6/1, Scope3/1
  Add11/1 -> Pr_gsc/1
  Multiply5/1 -> Add11/2
  Multiply4/1 -> Add11/1
  [Vsd] -> Multiply4/1
  [Vsq] -> Multiply5/1
  [Icd] -> Multiply4/2
  [Icq] -> Multiply5/2
  From14/1 -> Multiply2/1
  From12/1 -> Multiply2/2
  Multiply2/1 -> Add10/1
  From15/1 -> Multiply3/1
  From13/1 -> Multiply3/2
  Multiply3/1 -> Add10/2
  Add9/1 -> Add8/2
  Multiply1/1 -> Gain7/1
  [Icd] -> Multiply1/2
  Gain7/1 -> Add9/1
  [Vsq] -> Add9/2
  [We] -> Multiply1/1
  Gain6/1 -> KiIq_gw/1
  Gain5/1 -> Add7/1
  KiIq_gw/1 -> Add7/2
  Add7/1 -> Add8/1  "Vgq'"
  Constant1/1 -> Add6/1
  [Icq] -> Add6/2
  [Vsd] -> Add5/2
  Demux/1 -> [Vsd]
  Demux/2 -> [Vsq]
  Vsdq/1 -> Demux/1, [Vsdq]
  Add5/1 -> Add4/2
  Gain4/1 -> Add5/1
  [Icq] -> Multiply/2
  Multiply/1 -> Gain4/1
  [We] -> Multiply/1
  Add3/1 -> Add4/1  "Vgd'"
  Gain3/1 -> KiId_gw/1
  KiId_gw/1 -> Add3/2
  Add2/1 -> Gain2/1, Gain3/1, Scope4/1
  Gain2/1 -> Add3/1
  [Icd] -> Add2/2, Scope1/1
  Add1/1 -> Add2/1  "Iref_cd*"
  KiDC_gw/1 -> Add1/2
  Gain1/1 -> KiDC_gw/1
  Gain/1 -> Add1/1
  Add/1 -> Gain/1, Gain1/1
  [Vdc] -> Add/2
  Constant/1 -> Add/1
  Constant2/1 -> [We]
  Vdc/1 -> [Vdc]

== system M10B39_es_V3/Genrators/Wind Generator - DFIG2/Mechanical DE ==
  note: 这里是电动机惯例，因此发电的时候力矩应该是负的
  note: $\frac{d\omega_r}{dt}=\frac{1}{H}(T_e-T_m)$
      | 电动机惯例
  Te : Inport
  Tm : Inport  Port=2
  AWr : Integrator  InitialCondition=Wr0
  Add : Sum  Inputs=+-
  Constant2 : Constant
  Gain : Gain  Gain=1/H
  Scope : Scope
      settings: ActiveDisplayYMinimum=0.89006  ActiveDisplayYMaximum=0.98946
  Scope2 : Scope
      settings: ActiveDisplayYMinimum=-0.25  ActiveDisplayYMaximum=2.25  DataLoggingVariableName=ScopeData4
  Sum : Sum  Inputs=|-+
  "s " : Outport
  Wr : Outport  Port=2
  wires:
  Sum/1 -> "s "/1
  Tm/1 -> Scope2/1, Add/2
  Add/1 -> Gain/1
  Constant2/1 -> Sum/2
  Gain/1 -> AWr/1
  Te/1 -> Add/1
  AWr/1 -> Sum/1, Wr/1, Scope/1

== system M10B39_es_V3/Genrators/Wind Generator - DFIG2/NoIdealPLL ==
  note: $-V_{x}*sin(\delta_{pcc})+V_{y}*cos(\delta_{pcc})$
  Vsxy : Inport
  Add : Sum
  Add1 : Sum
  Constant : Constant
  Fcn1 : Fcn  Expr=sqrt(u(1)*u(1)+u(2)*u(2))
  Fcn3 : Fcn  Expr=u(1)*cos(u(3))+u(2)*sin(u(3))
  Fcn4 : Fcn  Expr=-u(1)*sin(u(3))+u(2)*cos(u(3))
  Gain : Gain  Gain=Kppll
  Gain1 : Gain  Gain=Kipll
  Integrator : Integrator
  Mux1 : Mux  Inputs=2
  Mux4 : Mux  Inputs=2
  PLL : Integrator  InitialCondition=Atheta
  Scope{,1..3} (4 alike) : Scope
      Scope settings: ActiveDisplayYMinimum=-0.99937  ActiveDisplayYMaximum=8.99437
      Scope1 settings: ActiveDisplayYMinimum=0.98212  ActiveDisplayYMaximum=1.13956
      Scope2 settings: ActiveDisplayYMinimum=0.98677  ActiveDisplayYMaximum=1.11907  DataLoggingVariableName=ScopeData2
      Scope3 settings: ActiveDisplayYMinimum=0.99657  ActiveDisplayYMaximum=1.01572
  low pass filter : simulink_extras/Additional Linear/Transfer Fcn (with initial outputs)  N=[1]  D="[1e-1  1]"  Y0=1  U0=1
  Vsdq : Outport
  Atheta : Outport  Port=2
  fw : Outport  Port=3
  wires:
  Fcn1/1 -> Scope3/1
  Add1/1 -> PLL/1, Add/1
  Fcn4/1 -> Mux1/2, Gain1/1, Gain/1
  Gain1/1 -> Integrator/1
  Integrator/1 -> Add1/2
  Gain/1 -> Add1/1
  low pass filter/1 -> fw/1, Scope2/1
  Add/1 -> low pass filter/1, Scope1/1
  Constant/1 -> Add/2
  Fcn3/1 -> Mux1/1
  Vsxy/1 -> Mux4/1
  Mux1/1 -> Vsdq/1, Fcn1/1
  Mux4/1 -> Fcn4/1, Fcn3/1
  PLL/1 -> Scope/1, Atheta/1, Mux4/2

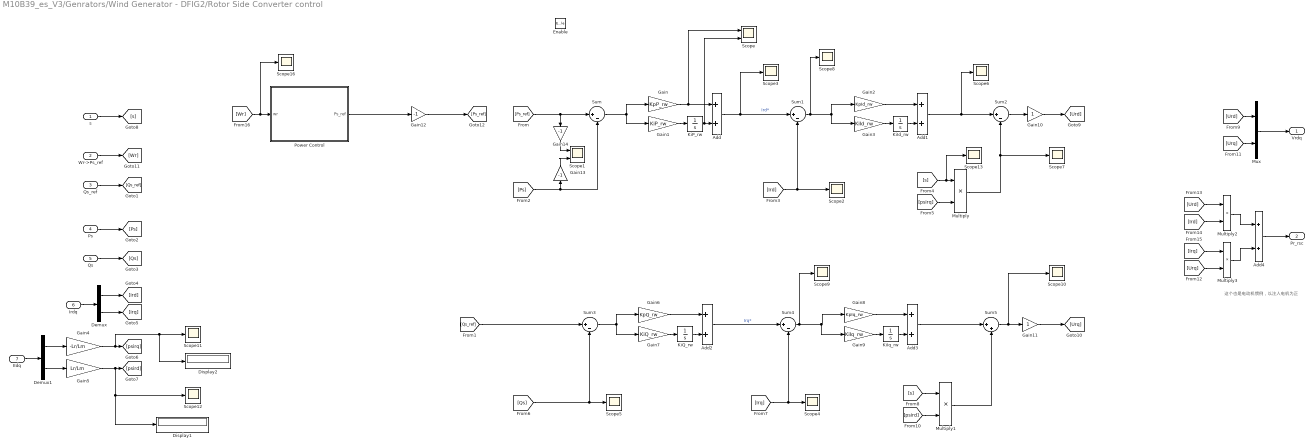
== system M10B39_es_V3/Genrators/Wind Generator - DFIG2/Rotor Side Converter control ==
  note: 这个也是电动机惯例，以注入电机为正
  s : Inport
  Wr->Ps_ref : Inport  Port=2
  Qs_ref : Inport  Port=3
  Ps : Inport  Port=4
  Qs : Inport  Port=5
  Irdq : Inport  Port=6
  Edq : Inport  Port=7
  Enable : EnablePort
  Add{,1..4} (5 alike) : Sum
  Demux : Demux  Outputs=2
  Demux1 : Demux  Outputs=2
  Display1 : Display
  Display2 : Display
  Gain : Gain  Gain=KpP_rw
  Gain1 : Gain  Gain=KiP_rw
  Gain10 : Gain
  Gain11 : Gain
  Gain12 : Gain  Gain=-1
  Gain13 : Gain  Gain=-1
  Gain14 : Gain  Gain=-1
  Gain2 : Gain  Gain=KpId_rw
  Gain3 : Gain  Gain=KiId_rw
  Gain4 : Gain  Gain=-Lr/Lm
  Gain5 : Gain  Gain=Lr/Lm
  Gain6 : Gain  Gain=KpQ_rw
  Gain7 : Gain  Gain=KiQ_rw
  Gain8 : Gain  Gain=KpIq_rw
  Gain9 : Gain  Gain=KiIq_rw
  KiId_rw : Integrator
  KiIq_rw : Integrator
  KiP_rw : Integrator  InitialCondition=Ird_ref
  KiQ_rw : Integrator  InitialCondition=Irq_ref
  Multiply{,1..3} (4 alike) : Product
  Mux : Mux  Inputs=2
  Power Control : Subsystem
  Scope : Scope  NumInputPorts=2
      settings: ActiveDisplayYMinimum=-0.15787  ActiveDisplayYMaximum=1.4048
  Scope1 : Scope  NumInputPorts=2
      settings: ActiveDisplayYMinimum=0.941157  ActiveDisplayYMaximum=0.94124  DataLoggingVariableName=ScopeData2
  Scope{2..13,16} (13 alike) : Scope
      Scope10 settings: ActiveDisplayYMinimum=-0.02713  ActiveDisplayYMaximum=0.00724  DataLoggingVariableName=ScopeData10
      Scope11 settings: DataLoggingVariableName=ScopeData13
      Scope12 settings: DataLoggingVariableName=ScopeData14
      Scope13 settings: ActiveDisplayYMinimum=-0.23407  ActiveDisplayYMaximum=0.19201  DataLoggingVariableName=ScopeData15
      Scope16 settings: ActiveDisplayYMinimum=-1.125  ActiveDisplayYMaximum=0.125  DataLoggingVariableName=ScopeData2
      Scope2 settings: ActiveDisplayYMinimum=0.9164  ActiveDisplayYMaximum=0.98721  DataLoggingVariableName=ScopeData4
      Scope3 settings: ActiveDisplayYMinimum=1.1610912356  ActiveDisplayYMaximum=1.1610912369  DataLoggingVariableName=ScopeData5
      Scope4 settings: ActiveDisplayYMinimum=-0.86275  ActiveDisplayYMaximum=6.60838  DataLoggingVariableName=ScopeData2
      Scope5 settings: ActiveDisplayYMinimum=-8E-13  ActiveDisplayYMaximum=6E-13  DataLoggingVariableName=ScopeData3
      Scope6 settings: ActiveDisplayYMinimum=0.00428  ActiveDisplayYMaximum=0.05974  DataLoggingVariableName=ScopeData2
      Scope7 settings: ActiveDisplayYMinimum=-0.10258  ActiveDisplayYMaximum=-0.10236  DataLoggingVariableName=ScopeData3
      Scope8 settings: ActiveDisplayYMinimum=-0.15319  ActiveDisplayYMaximum=1.32201  DataLoggingVariableName=ScopeData4
      Scope9 settings: ActiveDisplayYMinimum=-0.42548  ActiveDisplayYMaximum=0.04779  DataLoggingVariableName=ScopeData9
  Sum{,1..4} (5 alike) : Sum  Inputs=|+-
  Sum5 : Sum  Inputs=|++
  Vrdq : Outport
  Pr_rsc : Outport  Port=2
  wires:
  Gain12/1 -> [Ps_ref]
  Gain13/1 -> Scope1/2
  Gain14/1 -> Scope1/1
  [Qs_ref] -> Sum3/1
  Power Control/1(Ps_ref) -> Gain12/1
  [Wr] -> Power Control/1(wr), Scope16/1
  [Ird] -> Sum1/2, Scope2/1
  Add4/1 -> Pr_rsc/1
  Multiply3/1 -> Add4/2
  Multiply2/1 -> Add4/1
  [Urq] -> Multiply3/2
  [Irq] -> Multiply3/1
  [Ird] -> Multiply2/2
  [Urd] -> Multiply2/1
  KiP_rw/1 -> Add/2, Scope/2
  Gain/1 -> Add/1, Scope/1
  Gain11/1 -> [Urq]
  Gain10/1 -> [Urd]
  Mux/1 -> Vrdq/1
  [Urq] -> Mux/2
  [Urd] -> Mux/1
  Sum5/1 -> Gain11/1, Scope10/1
  Multiply1/1 -> Sum5/2
  [psird] -> Multiply1/2
  [s] -> Multiply1/1
  Add3/1 -> Sum5/1
  Gain9/1 -> KiIq_rw/1
  Sum4/1 -> Gain8/1, Gain9/1, Scope9/1
  Gain8/1 -> Add3/1
  KiIq_rw/1 -> Add3/2
  [Irq] -> Sum4/2, Scope4/1
  Gain7/1 -> KiQ_rw/1
  KiQ_rw/1 -> Add2/2
  Gain6/1 -> Add2/1
  Sum3/1 -> Gain6/1, Gain7/1
  Add2/1 -> Sum4/1  "Irq*"
  [Qs] -> Sum3/2, Scope5/1
  Sum2/1 -> Gain10/1
  Multiply/1 -> Sum2/2, Scope7/1
  [psirq] -> Multiply/2
  [s] -> Multiply/1, Scope13/1
  Gain5/1 -> [psird], Display1/1, Scope12/1
  Gain4/1 -> [psirq], Scope11/1, Display2/1
  Demux1/1 -> Gain4/1
  s/1 -> [s]
  Edq/1 -> Demux1/1
  Demux1/2 -> Gain5/1
  Gain3/1 -> KiId_rw/1
  KiId_rw/1 -> Add1/2
  Gain2/1 -> Add1/1
  Sum1/1 -> Gain2/1, Gain3/1, Scope8/1
  Add1/1 -> Sum2/1, Scope6/1
  Add/1 -> Scope3/1, Sum1/1  "Ird*"
  Sum/1 -> Gain/1, Gain1/1
  Gain1/1 -> KiP_rw/1
  [Ps] -> Gain13/1, Sum/2
  [Ps_ref] -> Sum/1, Gain14/1
  Demux/2 -> [Irq]
  Demux/1 -> [Ird]
  Irdq/1 -> Demux/1
  Qs/1 -> [Qs]
  Ps/1 -> [Ps]
  Qs_ref/1 -> [Qs_ref]
  Wr->Ps_ref/1 -> [Wr]

== system M10B39_es_V3/Genrators/Wind Generator - DFIG2/Wind Turbine ==
  note: $C_p=0.22* \lbrack 116*(\frac{1}{\lambda+0.008\beta}-\frac{0.0035}{\beta^3+1})-0.48\beta-5 \rbrack * e^{-12.5*(\frac{1}{\lambda+0.08\beta}-\frac{0.035}{\beta^3+1}) }$
  note: $P_m=0.95*\frac{1.2}{(12^3*0.5)}*\lbrack 43.268*(\frac{v_w}{99.4945*\omega_r}-0.035)-1.865 \rbrack * e^{-12.5*(\frac{v_w}{99.4945*\omega_r}-0.035) }*v_w^3$
  note: $C_p= \lbrack 43.268*(\frac{v_w}{99.4945*\omega_r}-0.035)-1.865 \rbrack * e^{-12.5*(\frac{v_w}{99.4945*\omega_r}-0.035) }$
  note: $P_m=0.95*\frac{1.2}{(12^3*0.5)}*\lbrack 43.268*(\frac{1}{99.4945*\frac{\omega_r}{v_w}}-0.035)-1.865 \rbrack * e^{-12.5*(\frac{1}{99.4945*\frac{\omega_r}{v_w}}-0.035) }*v_w^3$
  note: $C_p= \lbrack 43.268*(\frac{1}{99.4945*\frac{\omega_r}{v_w}}-0.035)-1.865 \rbrack * e^{-12.5*(\frac{1}{99.4945*\frac{\omega_r}{v_w}}-0.035) }$
  note: $P_m=0.95*\frac{1.2}{(12^3*0.5)}*C_p*v_w^3$
  note: $C_p= \lbrack 43.268*(\frac{1}{\lambda}-0.035)-1.865 \rbrack * e^{-12.5*(\frac{1}{\lambda}-0.035) }$
  note: $C_p=0.373* \lbrack 116*(\frac{1}{\lambda}-0.035)-5 \rbrack * e^{-12.5*(\frac{1}{\lambda}-0.035) }$
  note: 叶片旋转角速度
  note: 风力机输出
      | 的机械功率
  note: 叶尖速比
  note: 风能利用系数与桨矩角
      | 和叶尖速比之间的关系
  note: 风能利用
      | 系数
  note: 风力机输出
      | 的机械功率
  note: 风速
  note: 叶片旋转速度
  note: 考虑了机械损耗
  note: $\lambda=99.4945*\frac{\omega_r}{v_w}$
  note: $C_p=0.373* \lbrack 116*(\frac{1}{\lambda+0.08\beta}-\frac{0.035}{\beta^3+1})-0.4\beta-5 \rbrack * e^{-12.5*(\frac{1}{\lambda+0.08\beta}-\frac{0.035}{\beta^3+1}) }$
  note: $P_m=\frac{1.2}{(12^3*0.5)}*C_p*v_w^3$
  note: J. Chen and D. Jiang, "Study on modeling and simulation of non-grid-connected wind turbine," 2009 World Non-Grid-Connected Wind Power and Energy Conference , Nanjing, 2009, pp. 1-5. doi: 10.1109/WNWEC.2009.5335791
  W_wt (pu) : Inport
  Pitch angle (deg) : Inport  Port=2
  Wind speed (m/s) : Inport  Port=3
  ->pu1 : Gain  Gain=0.95
  ->pu2 : Gain  Gain=0.95
  Avoid div. by zero : Saturate  UpperLimit=inf  LowerLimit=eps
  "Avoid div. by zero " : Saturate  UpperLimit=inf  LowerLimit=eps
  Display2 : Display
  Fcn2 : Fcn  Expr=99.4945*u[2]/u[1]
  Fcn4 : Fcn  Expr=0.22*(116*(1/(u(1)+0.008*u(2))-0.0035/((u(2)^3)+1))-0.48*u(2)-5)*exp(-12.5*(1/(u(1)+0.008*u(2))-0.0035/((u(2)^3)+1)))
  "K2*Cp*wind^3 " : Fcn  Expr=1.2/(12^3*0.5)*u[1]^3*u[2]
  Mux : Mux  Inputs=2
  Mux1 : Mux  Inputs=2
  Mux2 : Mux  Inputs=2
  Product2 : Product  Inputs=*/  InputSameDT=on  SaturateOnIntegerOverflow=on  OutDataTypeStr=Inherit: Same as first input
  Scope{1..3,5} (4 alike) : Scope
      Scope1 settings: ActiveDisplayYMinimum=6.3327  ActiveDisplayYMaximum=6.33385  DataLoggingSaveFormat=Array
      Scope2 settings: ActiveDisplayYMinimum=0.10425  ActiveDisplayYMaximum=1.46932  DataLoggingVariableName=ScopeData25
      Scope3 settings: ActiveDisplayYMinimum=0.5999  ActiveDisplayYMaximum=0.6001  DataLoggingVariableName=Pw  DataLoggingSaveFormat=Array
      Scope5 settings: ActiveDisplayYMinimum=0.64296  ActiveDisplayYMaximum=0.84296  DataLoggingVariableName=Pw2  DataLoggingSaveFormat=Array
  Subsystem : Subsystem  Commented=on
  Tm : Outport
  Pm : Outport  Port=2
  wires:
  ->pu2/1 -> Pm/1
  Fcn4/1 -> Scope5/1, Mux2/2
  "K2*Cp*wind^3 "/1 -> Scope3/1, Display2/1, Product2/1, ->pu2/1
  Wind speed (m/s)/1 -> Avoid div. by zero/1
  Product2/1 -> ->pu1/1
  ->pu1/1 -> Scope2/1, Tm/1
  W_wt (pu)/1 -> "Avoid div. by zero "/1
  "Avoid div. by zero "/1 -> Product2/2, Mux/2
  Avoid div. by zero/1 -> Mux2/1, Mux/1
  Pitch angle (deg)/1 -> Mux1/2
  Mux2/1 -> "K2*Cp*wind^3 "/1
  Mux/1 -> Fcn2/1
  Mux1/1 -> Fcn4/1
  Fcn2/1 -> Mux1/1, Scope1/1  "lambda"

== system M10B39_es_V3/Genrators/Wind Generator - DFIG2/dq-xy ==
  dq : Inport
  delta_xy : Inport  Port=2
  Complex to Magnitude-Angle : ComplexToMagnitudeAngle
  Demux : Demux  Outputs=2
  Fcn3 : Fcn  Expr=u(1)*cos(u(2))
  Fcn4 : Fcn  Expr=u(1)*sin(u(2))
  Mux1 : Mux  Inputs=2
  Mux2 : Mux  Inputs=2
  Real-Imag to Complex : RealImagToComplex
  Scope : Scope
      settings: ActiveDisplayYMinimum=0.298155365983  ActiveDisplayYMaximum=0.298155366015  DataLoggingVariableName=ScopeData2
  Scope1 : Scope  NumInputPorts=2
      settings: ActiveDisplayYMinimum=1.04058  ActiveDisplayYMaximum=1.12593  DataLoggingVariableName=ScopeData51  DataLoggingSaveFormat=Array
  Scope2 : Scope  NumInputPorts=2
      settings: ActiveDisplayYMinimum=1.01502  ActiveDisplayYMaximum=1.10979  DataLoggingVariableName=ScopeData56  DataLoggingSaveFormat=Array
  Sum14 : Sum  Inputs=|++
  xy : Outport
  wires:
  Mux2/1 -> xy/1
  dq/1 -> Demux/1
  Demux/2 -> Real-Imag to Complex/2
  Demux/1 -> Real-Imag to Complex/1
  Real-Imag to Complex/1 -> Complex to Magnitude-Angle/1
  delta_xy/1 -> Sum14/2
  Fcn3/1 -> Mux2/1, Scope2/1
  Fcn4/1 -> Scope2/2, Mux2/2
  Mux1/1 -> Fcn3/1, Fcn4/1
  Complex to Magnitude-Angle/2 -> Sum14/1, Scope/1
  Complex to Magnitude-Angle/1 -> Mux1/1, Scope1/1
  Sum14/1 -> Mux1/2, Scope1/2

== system M10B39_es_V3/Genrators/Wind Generator - DFIG2/dq-xy1 ==
  dq : Inport
  delta_xy : Inport  Port=2
  Complex to Magnitude-Angle : ComplexToMagnitudeAngle
  Demux : Demux  Outputs=2
  Fcn3 : Fcn  Expr=u(1)*cos(u(2))
  Fcn4 : Fcn  Expr=u(1)*sin(u(2))
  Mux1 : Mux  Inputs=2
  Mux2 : Mux  Inputs=2
  Real-Imag to Complex : RealImagToComplex
  Scope : Scope
      settings: ActiveDisplayYMinimum=0.298155365983  ActiveDisplayYMaximum=0.298155366015  DataLoggingVariableName=ScopeData2
  Scope1 : Scope  NumInputPorts=2
      settings: ActiveDisplayYMinimum=1.04058  ActiveDisplayYMaximum=1.12593  DataLoggingVariableName=ScopeData51  DataLoggingSaveFormat=Array
  Scope2 : Scope  NumInputPorts=2
      settings: ActiveDisplayYMinimum=1.01502  ActiveDisplayYMaximum=1.10979  DataLoggingVariableName=ScopeData56  DataLoggingSaveFormat=Array
  Sum14 : Sum  Inputs=|++
  xy : Outport
  wires:
  Mux2/1 -> xy/1
  dq/1 -> Demux/1
  Demux/2 -> Real-Imag to Complex/2
  Demux/1 -> Real-Imag to Complex/1
  Real-Imag to Complex/1 -> Complex to Magnitude-Angle/1
  delta_xy/1 -> Sum14/2
  Fcn3/1 -> Mux2/1, Scope2/1
  Fcn4/1 -> Scope2/2, Mux2/2
  Mux1/1 -> Fcn3/1, Fcn4/1
  Complex to Magnitude-Angle/2 -> Sum14/1, Scope/1
  Complex to Magnitude-Angle/1 -> Mux1/1, Scope1/1
  Sum14/1 -> Mux1/2, Scope1/2
